simulink model "Example_3_Closed"  (Simulink 8.3)
settings: Solver=ode45  StartTime=0.0  StopTime=60  RelTol=1e-3
settings Model: Creator=NeuControl  LastModifiedBy=Li Jinghao
settings DataIOCC: SignalLoggingSaveFormat=Dataset
settings DebuggingCC: UnderspecifiedInitializationDetection=Simplified  StateNameClashWarn=none
settings GRTTargetCC: CombineOutputUpdateFcns=on  GRTInterface=off

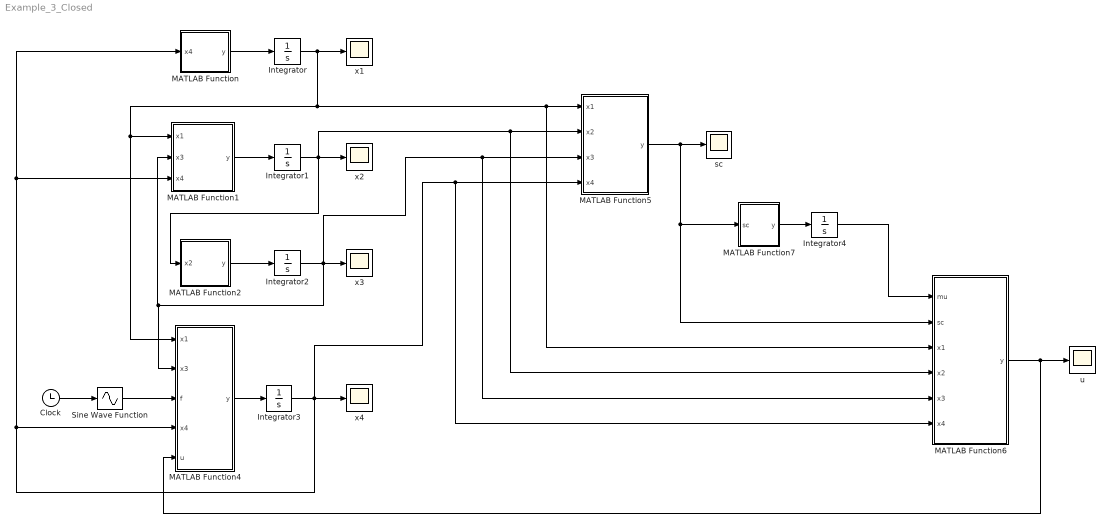
== system Example_3_Closed ==
  Clock : Clock
  Integrator : Integrator  InitialCondition=pi/6
  Integrator{1..4} (4 alike) : Integrator
  MATLAB Function : MATLAB Function  TreatAsAtomicUnit=on
  MATLAB Function1 : MATLAB Function  TreatAsAtomicUnit=on
  MATLAB Function2 : MATLAB Function  TreatAsAtomicUnit=on
  MATLAB Function4 : MATLAB Function  TreatAsAtomicUnit=on
  MATLAB Function5 : MATLAB Function  TreatAsAtomicUnit=on
  MATLAB Function6 : MATLAB Function  TreatAsAtomicUnit=on
  MATLAB Function7 : MATLAB Function  TreatAsAtomicUnit=on
  Sine Wave Function : Sin  TimeSource=Use external signal  SampleTime=0
  sc : Scope
      settings: SaveName=s
  u : Scope
      settings: SaveName=u
  x{1..4} (4 alike) : Scope
      x1 settings: SaveName=x1
      x2 settings: SaveName=x2
      x3 settings: SaveName=x3
      x4 settings: SaveName=x4
  wires:
  Integrator/1 -> MATLAB Function4/1(x1), MATLAB Function1/1(x1), MATLAB Function6/3(x1), MATLAB Function5/1(x1), x1/1
  MATLAB Function/1(y) -> Integrator/1
  MATLAB Function1/1(y) -> Integrator1/1
  Integrator1/1 -> MATLAB Function6/4(x2), MATLAB Function5/2(x2), MATLAB Function2/1(x2), x2/1
  Integrator2/1 -> MATLAB Function6/5(x3), MATLAB Function5/3(x3), MATLAB Function4/2(x3), MATLAB Function1/2(x3), x3/1
  MATLAB Function2/1(y) -> Integrator2/1
  MATLAB Function4/1(y) -> Integrator3/1
  Integrator3/1 -> MATLAB Function6/6(x4), MATLAB Function5/4(x4), x4/1, MATLAB Function/1(x4), MATLAB Function1/3(x4), MATLAB Function4/4(x4)
  Sine Wave Function/1 -> MATLAB Function4/3(f)
  Clock/1 -> Sine Wave Function/1
  MATLAB Function5/1(y) -> MATLAB Function7/1(sc), MATLAB Function6/2(sc), sc/1
  MATLAB Function6/1(y) -> MATLAB Function4/5(u), u/1
  MATLAB Function7/1(y) -> Integrator4/1
  Integrator4/1 -> MATLAB Function6/1(mu)

== matlab function MATLAB Function1 ==
  data: x1 input double; x3 input double; x4 input double; y output double
function y = fcn(x1,x3,x4)
%#codegen

m=2;
M=8;
l=0.5;

y = x3-(m*l/(m+M))*cos(x1)*x4;

== matlab function MATLAB Function ==
  data: x4 input double; y output double
function y = fcn(x4)
%#codegen

y = x4;

== matlab function MATLAB Function2 ==
  data: x2 input double; y output double
function y = fcn(x2)
%#codegen

m=2;
M=8;
k=0.5;
y = -(k/(m+M))*x2;

== matlab function MATLAB Function4 ==
  data: x1 input double; x3 input double; f input double; x4 input double; y output double; u input double
function y = fcn(x1,x3,f,x4,u)
%#codegen

m=2;
M=8;
l=0.5;
k=0.5;
y = 1/(4/3*m*l*l*(m+M)-m*m*l*l*cos(x1)*cos(x1))...
    *(-m*m*l*l*sin(x1)*cos(x1)*x4+k*m*l*cos(x1)*x3+(m+M)*(u+f));

== matlab function MATLAB Function5 ==
  data: x1 input double; x2 input double; x3 input double; x4 input double; y output double
function y = fcn(x1,x2,x3,x4)
%#codegen

Sc=[7.1868   32.9483  615.9913];
x=[x1;x2;x3];
y = Sc*x+x4;

== matlab function MATLAB Function6 ==
  data: mu input double; sc input double; x1 input double; x2 input double; x3 input double; x4 input double; y output double
function y = fcn(mu,sc,x1,x2,x3,x4)
%#codegen

m=2;
M=8;
l=0.5;
k=0.5;
xi=pi/3;
a=cos(xi);
v1=(cos(x1)-a)/(1-a);
v2=(1-cos(x1))/(1-a);
Sc=[7.1868   32.9483  615.9913];
A11=[0 0 0;0 0 1;0 -k/(m+M) 0];
A21=[0 0 0;0 0 1;0 -k/(m+M) 0];
A12=[1;-m*l/(m+M);0];
A22=[1;-a*m*l/(m+M);0];
A1=v1*A11+v2*A21;
A2=v1*A12+v2*A22;
x=[x1;x2;x3];
B1=4/3*m*l*l*(m+M)-m*m*l*l*cos(x1)*cos(x1);
kappa=0.5;
delta=0.001;
beta=10;
epsilon=0.1;
bdf=1;
bx4=3;
rho=(m+M)/(4/3*m*l*l*(m+M)-m*m*l*l)*bdf+2*(m+M)*m*m*l*l*bx4/((4/3*m*l*l*(m+M)-m*m*l*l)*(4/3*m*l*l*(m+M)-m*m*l*l));
k1=delta+1/beta*(rho*rho/(4*epsilon)+2*epsilon*rho+epsilon+2*epsilon*beta+8*epsilon^3);
k2=beta+4*epsilon^2+2*epsilon*k1;
k3=1;

y = -1/(m+M)*B1*((Sc*A1*x+1/B1*k*m*l*cos(x1)*x2+kappa*Sc*x)+(Sc*A2*x4-1/B1*m*m*l*l*sin(x1)*cos(x1)*x4*x4+kappa*x4)++k1*(sc/sqrt(norm(sc))+k3*sc)-mu);

== matlab function MATLAB Function7 ==
  data: sc input double; y output double
function y = fcn(sc)
%#codegen

m=2;
M=8;
l=0.5;
delta=0.001;
beta=10;
epsilon=0.1;
bdf=1;
bx4=3;
rho=(m+M)/(4/3*m*l*l*(m+M)-m*m*l*l)*bdf...
    +2*(m+M)*m*m*l*l*bx4/((4/3*m*l*l*(m+M)-m*m*l*l)*(4/3*m*l*l*(m+M)-m*m*l*l));
k1=delta+1/beta*(rho*rho/(4*epsilon)+2*epsilon*rho+epsilon+2*epsilon*beta+8*epsilon^3);
k2=beta+4*epsilon^2+2*epsilon*k1;
k3=1;

y = -k2*(1/2*sc/norm(sc)+3/2*k3*sc/sqrt(norm(sc))+k3^2*sc);
